simulink model "ModeStateCtrlCaller"  (R2018b)
settings: Solver=FixedStepDiscrete  StartTime=0.0  StopTime=10.0  RelTol=1e-3
undefined symbols (not defined in the file or in its folder): MdSWReqChk_Cal, MdXX_QuitChk_Cal, MdXXArray_Cal, modestate32
settings Model: Creator=sn2xws  LastModifiedBy=sn2xws
settings DataIOCC: SaveFormat=StructureWithTime
settings OptimizationCC: DefaultParameterBehavior=Inlined  EnhancedBackFolding=on  PassReuseOutputArgsAs=Individual arguments  ZeroExternalMemoryAtStartup=off  ZeroInternalMemoryAtStartup=off  OptimizeBlockOrder=speed  DifferentSizesBufferReuse=on  OptimizationCustomize=off
settings DebuggingCC: ParameterTunabilityLossMsg=error
settings SFSimCC: MATLABDynamicMemAlloc=off
settings RTWCC: SystemTargetFile=autosar.tlc  GenCodeOnly=on  TemplateMakefile=ert_default_tmf  Description=AUTOSAR  GenerateReport=on  IncludeHyperlinkInReport=on  LaunchReport=on  GenerateTraceInfo=on  GenerateTraceReport=on  GenerateTraceReportSl=on  GenerateTraceReportSf=on  GenerateTraceReportEml=on  GenerateCodeMetricsReport=on
settings CodeAppCC: ForceParamTrailComments=on  IgnoreCustomStorageClasses=off  OperatorAnnotations=on  SimulinkDataObjDesc=on  SFDataObjDesc=on  InsertBlockDesc=on
settings STFCustomTargetCC: TargetLangStandard=C99 (ISO)  MultiwordLength=256  ParMdlRefBuildCompliant=on  CompOptLevelCompliant=on  IncludeMdlTerminateFcn=off  CombineOutputUpdateFcns=on  SuppressErrorStatus=on  ERTCustomFileBanners=on  SupportNonFinite=off  SupportComplex=off  SupportContinuousTime=off  SupportNonInlinedSFcns=off  RemoveResetFunc=on  MATLABClassNameForMDSCustomization=Simulink.SoftwareTarget.ERTCustomization  AutosarCompliant=on  UseToolchainInfoCompliant=on  LookupTableObjectStructAxisOrder=2,1,3,4,...  LUTObjectStructOrderEvenSpacing=Size,Table,Breakpoints  SystemTargetFile=autosar.tlc
settings ERTTargetCC: TargetLangStandard=C99 (ISO)  ConcurrentExecutionCompliant=off  IncludeMdlTerminateFcn=off  SuppressErrorStatus=on  SupportNonFinite=off  SupportComplex=off  ModelStepFunctionPrototypeControlCompliant=off  CPPClassGenCompliant=off  AutosarCompliant=on  LookupTableObjectStructAxisOrder=2,1,3,4,...  LUTObjectStructOrderEvenSpacing=Size,Table,Breakpoints  InlinedParameterPlacement=NonHierarchical  ERTCustomFileTemplate=example_file_process.tlc  ERTFilePackagingFormat=Compact

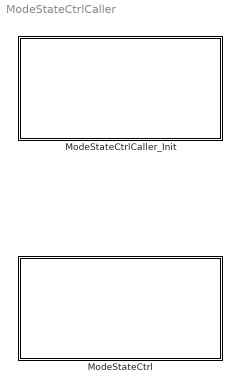
== system ModeStateCtrlCaller ==
  ModeStateCtrl : Subsystem
  ModeStateCtrlCaller_Init : Subsystem

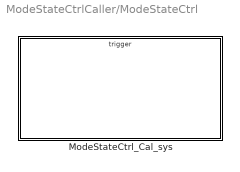
== system ModeStateCtrlCaller/ModeStateCtrl ==
  ModeStateCtrl_Cal_sys : Subsystem

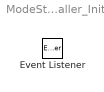
== system ModeStateCtrlCaller/ModeStateCtrlCaller_Init ==
  Event Listener : EventListener  EventName=reset

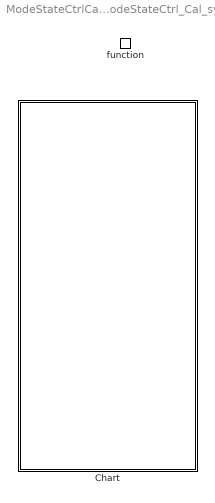
== system ModeStateCtrlCaller/ModeStateCtrl/ModeStateCtrl_Cal_sys ==
  function : TriggerPort  TriggerType=function-call  IsSimulinkFunction=on  FunctionName=ModeStateCtrl_Cal  VariantControl=(inherit)
  Chart : Stateflow chart  TreatAsAtomicUnit=on

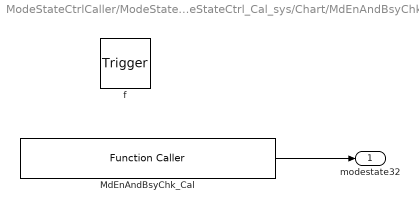
== system ModeStateCtrlCaller/ModeStateCtrl/ModeStateCtrl_Cal_sys/Chart/MdEnAndBsyChk_Cal ==
  f : TriggerPort  TriggerType=function-call  VariantControl=(inherit)
      settings: CopyFcn=Stateflow.SLINSF.SimulinkMan.removeBlockPreDeleteFcn  PreDeleteFcn=Stateflow.SLINSF.SimulinkMan.unsafePredeleteFcn
  MdEnAndBsyChk_Cal : FunctionCaller  FunctionPrototype=modestate32 = MdEnAndBsyChk_Cal()  OutputArgumentSpecifications=uint32(1)
  modestate32 : Outport
  wires:
  MdEnAndBsyChk_Cal/1 -> modestate32/1

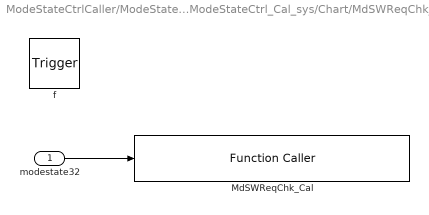
== system ModeStateCtrlCaller/ModeStateCtrl/ModeStateCtrl_Cal_sys/Chart/MdSWReqChk_Cal ==
  modestate32 : Inport  OutDataTypeStr=uint32  PortDimensions=1
  f : TriggerPort  TriggerType=function-call  VariantControl=(inherit)
      settings: CopyFcn=Stateflow.SLINSF.SimulinkMan.removeBlockPreDeleteFcn  PreDeleteFcn=Stateflow.SLINSF.SimulinkMan.unsafePredeleteFcn
  MdSWReqChk_Cal : FunctionCaller  FunctionPrototype=MdSWReqChk_Cal(modestate32)  InputArgumentSpecifications=uint32(1)
  wires:
  modestate32/1 -> MdSWReqChk_Cal/1

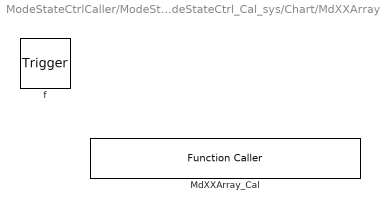
== system ModeStateCtrlCaller/ModeStateCtrl/ModeStateCtrl_Cal_sys/Chart/MdXXArray_Cal ==
  f : TriggerPort  TriggerType=function-call  VariantControl=(inherit)
      settings: CopyFcn=Stateflow.SLINSF.SimulinkMan.removeBlockPreDeleteFcn  PreDeleteFcn=Stateflow.SLINSF.SimulinkMan.unsafePredeleteFcn
  MdXXArray_Cal : FunctionCaller  FunctionPrototype=MdXXArray_Cal()

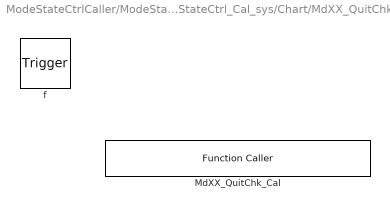
== system ModeStateCtrlCaller/ModeStateCtrl/ModeStateCtrl_Cal_sys/Chart/MdXX_QuitChk_Cal ==
  f : TriggerPort  TriggerType=function-call  VariantControl=(inherit)
      settings: CopyFcn=Stateflow.SLINSF.SimulinkMan.removeBlockPreDeleteFcn  PreDeleteFcn=Stateflow.SLINSF.SimulinkMan.unsafePredeleteFcn
  MdXX_QuitChk_Cal : FunctionCaller  FunctionPrototype=MdXX_QuitChk_Cal()

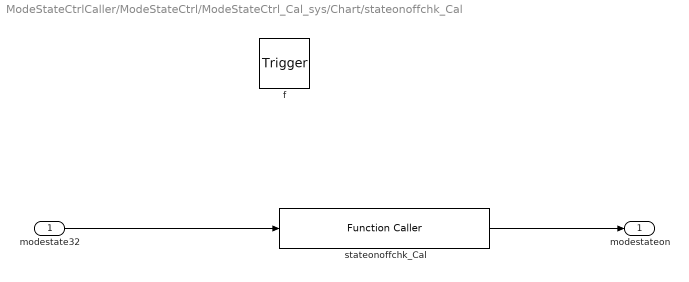
== system ModeStateCtrlCaller/ModeStateCtrl/ModeStateCtrl_Cal_sys/Chart/stateonoffchk_Cal ==
  modestate32 : Inport  OutDataTypeStr=uint32  PortDimensions=1
  f : TriggerPort  TriggerType=function-call  VariantControl=(inherit)
      settings: CopyFcn=Stateflow.SLINSF.SimulinkMan.removeBlockPreDeleteFcn  PreDeleteFcn=Stateflow.SLINSF.SimulinkMan.unsafePredeleteFcn
  stateonoffchk_Cal : FunctionCaller  FunctionPrototype=modestateon = stateonoffchk_Cal(modestate32)  InputArgumentSpecifications=uint32(1)  OutputArgumentSpecifications=boolean(true)
  modestateon : Outport
  wires:
  modestate32/1 -> stateonoffchk_Cal/1
  stateonoffchk_Cal/1 -> modestateon/1

== stateflow chart ModeStateCtrlCaller/ModeStateCtrl/ModeStateCtrl_Cal_sys/Chart ==
  state modestateon = stateonoffchk_Cal(modestate32) [function]
  state MdXXArray_Cal [function]
  state MdXX_QuitChk_Cal [function]
  state MdSWReqChk_Cal(modestate32) [function]
  state modestate32 = MdEnAndBsyChk_Cal [function]
  (default) -> (junction 2)
  (junction 2) -> (junction 28) [order 1] : [IsFirstTime]
  (junction 2) -> (junction 32) [order 2]
  (junction 28) -> (junction 30) : {
      | modestate32=uint32(0);
      | IsFirstTime = false;
      | }
  (junction 30) -> (junction 32)
  (junction 32) -> (junction 4) : {
      | modestateon = stateonoffchk_Cal(modestate32);
      | }
  (junction 4) -> (junction 17) [order 1] : [modestateon]
  (junction 4) -> (junction 21) [order 2] : {modestate32 = 0;}
  (junction 17) -> (junction 19) : {
      | MdXXArray_Cal();
      | MdXX_QuitChk_Cal();
      | MdSWReqChk_Cal(modestate32);
      | modestate32 = MdEnAndBsyChk_Cal();
      | }
  (junction 19) -> (junction 21)
  (junction 21) -> (junction 24)
  data: modestate32 function_input uint32 size=1; modestateon function_output; modestate32 function_input uint32 size=1; modestate32 function_output; modestateon local boolean; modestate32 local uint32; IsFirstTime local boolean =true
